simulink model "Automatic_Movement"  (R2015a)
settings: Solver=ode45  StartTime=0.0  StopTime=inf  FixedStep=0.05  RelTol=1e-3
values from neighbouring files (symbols this model uses):
  a_1 = 10.2    [Parameters.m]
  a_2 = 13.1    [Parameters.m]
  a_3 = 5.5    [Parameters.m]
  a_4 = 17    [Parameters.m]
  a_5 = 16.5    [Parameters.m]
  b_1 = 0.243    [Parameters.m]
  b_2 = 0.175    [Parameters.m]
  b_3 = 0.14    [Parameters.m]
  b_4 = 0.14    [Parameters.m]
  b_5 = 0.15    [Parameters.m]
  k1_1 = 2*alpha-a_1    (= 13.8)    [Parameters.m]
  k1_2 = 2*alpha-a_2    (= 10.9)    [Parameters.m]
  k1_3 = 2*alpha-a_3    (= 18.5)    [Parameters.m]
  k1_4 = 2*alpha-a_4    (= 7)    [Parameters.m]
  k1_5 = 2*alpha-a_5    (= 7.5)    [Parameters.m]
  k2_1 = alpha^2-b_1*k1_1    (= 140.6466)    [Parameters.m]
  k2_2 = alpha^2-b_2*k1_2    (= 142.0925)    [Parameters.m]
  k2_3 = alpha^2-b_3*k1_3    (= 141.41)    [Parameters.m]
  k2_4 = alpha^2-b_4*k1_4    (= 143.02)    [Parameters.m]
  k2_5 = alpha^2-b_5*k1_5    (= 142.875)    [Parameters.m]
  Ts = 0.06    [Parameters.m]
  Va = 24    [Parameters.m]
undefined symbols (not defined in the file or in its folder): DiscIntNeverNeededParam, gray, none, strel, videoinput
libraries: simulink x33, arduino_io_lib x28, visiontextngfix x6, visionanalysis x6, visionmorphops x4, visionstatistics x2, visionsinks x2, imaqlib x1
(part 1 of 2)
settings Model: CovMetricSettings=dwe  CovHtmlReporting=off  covSaveCumulativeToWorkspaceVar=off  CovSaveSingleToWorkspaceVar=off  CovExternalEMLEnable=on  ExtModeTrigDuration=10000  Creator=Antonio  LastModifiedBy=Antonio
settings SolverCC: PositivePriorityOrder=on
settings DataIOCC: LimitDataPoints=off  SaveFormat=Dataset
settings DebuggingCC: SFUnexpectedBacktrackingDiag=error  SFNoUnconditionalDefaultTransitionDiag=error
settings HardwareCC: ProdBitPerPointer=64  ProdLargestAtomicFloat=Float  ProdIntDivRoundTo=Zero  ProdEndianess=LittleEndian  ProdHWDeviceType=Specified
settings ModelReferenceCC: PropagateSignalLabelsOutOfModel=on
settings RTWCC: SystemTargetFile=quarc_win64.tlc  TemplateMakefile=quarc_default_tmf  Description=QUARC Win64 Target
settings STFCustomTargetCC: TargetLibSuffix=.lib  TargetPreCompLibLocation=C:\PROGRA~3\QUARC\lib\2017a\win64\release  TargetLangStandard=C99 (ISO)  GenerateSampleERTMain=off  ConcurrentExecutionCompliant=on  ERTCustomFileBanners=off  SupportNonInlinedSFcns=on  SupportVariableSizeSignals=off  MATLABClassNameForMDSCustomization=Simulink.SoftwareTarget.GRTCustomization  GRTInterface=on  SystemTargetFile=quarc_win64.tlc
settings GRTTargetCC: TargetPreCompLibLocation=C:\PROGRA~3\QUARC\lib\2017a\win64\release  TargetLangStandard=C99 (ISO)  ParMdlRefBuildCompliant=off  CompOptLevelCompliant=off  GeneratePreprocessorConditionals=Use local settings  CombineOutputUpdateFcns=off  MatFileLogging=off  CPPClassGenCompliant=off  GRTInterface=on  ExtMode=on  ExtModeMexFile=quarc_comm

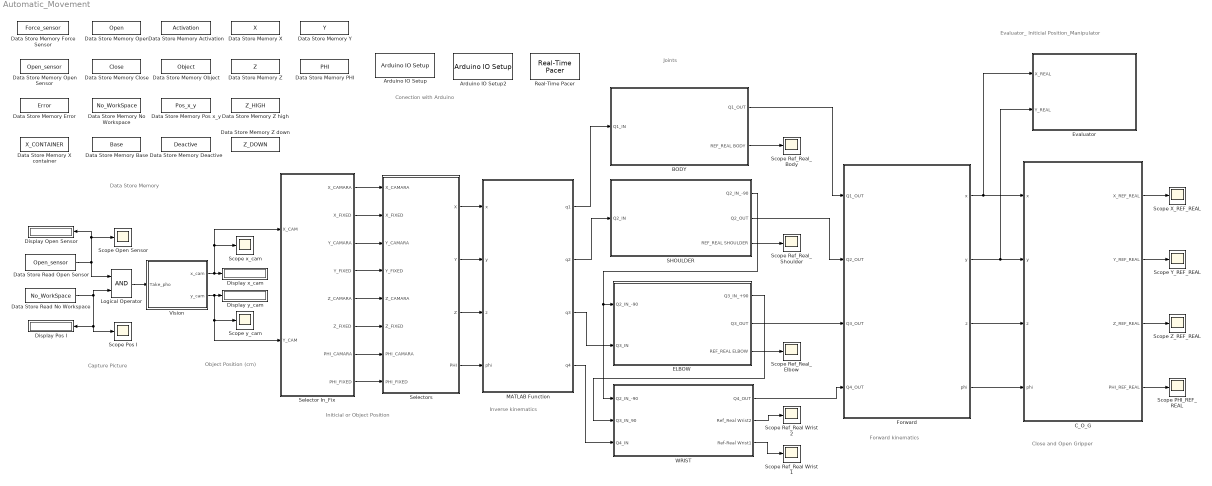
== system Automatic_Movement ==
  note: Close and Open Gripper
  note: Forward kinematics
  note: Joints
  note: Inverse kinematics
  note: Initicial or Object Position
  note: Evaluator_ Initicial Position_Manipulator
  note: Object Position
      | (cm)
  note: Capture Picture
  note: Data Store Memory
  note: Conection with Arduino
  Arduino IO Setup : arduino_io_lib/Arduino IO Setup  Priority=3  arduinoVar=Temporary arduino variable: Arduino1  workspaceVarName=a  comPort=COM3
  Arduino IO Setup2 : arduino_io_lib/Arduino IO Setup  Priority=3  arduinoVar=Temporary arduino variable: Arduino2  workspaceVarName=a  comPort=COM9
  BODY : Subsystem
  C_O_G : Subsystem
  Data Store Memory Base : DataStoreMemory  DataStoreName=Base  ReadBeforeWriteMsg=warning  WriteAfterWriteMsg=warning  WriteAfterReadMsg=warning  ShowAdditionalParam=off
  Data Store Memory Deactive : DataStoreMemory  DataStoreName=Deactive  ReadBeforeWriteMsg=warning  WriteAfterWriteMsg=warning  WriteAfterReadMsg=warning  ShowAdditionalParam=off
  Data Store Memory PHI : DataStoreMemory  DataStoreName=PHI  ReadBeforeWriteMsg=warning  WriteAfterWriteMsg=warning  WriteAfterReadMsg=warning  ShowAdditionalParam=off
  Data Store Memory Pos x_y : DataStoreMemory  DataStoreName=Pos_x_y  ReadBeforeWriteMsg=warning  WriteAfterWriteMsg=warning  WriteAfterReadMsg=warning  ShowAdditionalParam=off
  Data Store Memory Z : DataStoreMemory  DataStoreName=Z  ReadBeforeWriteMsg=warning  WriteAfterWriteMsg=warning  WriteAfterReadMsg=warning  ShowAdditionalParam=off
  Data Store Memory Z down : DataStoreMemory  DataStoreName=Z_DOWN  ReadBeforeWriteMsg=warning  WriteAfterWriteMsg=warning  WriteAfterReadMsg=warning  ShowAdditionalParam=off
  Data Store Memory Activation : DataStoreMemory  DataStoreName=Activation  ReadBeforeWriteMsg=warning  WriteAfterWriteMsg=warning  WriteAfterReadMsg=warning  ShowAdditionalParam=off
  "Data Store Memory Close " : DataStoreMemory  DataStoreName=Close  ReadBeforeWriteMsg=warning  WriteAfterWriteMsg=warning  WriteAfterReadMsg=warning  ShowAdditionalParam=off
  Data Store Memory Error : DataStoreMemory  DataStoreName=Error  ReadBeforeWriteMsg=warning  WriteAfterWriteMsg=warning  WriteAfterReadMsg=warning  ShowAdditionalParam=off
  Data Store Memory Force Sensor : DataStoreMemory  DataStoreName=Force_sensor  ReadBeforeWriteMsg=warning  WriteAfterWriteMsg=warning  WriteAfterReadMsg=warning  ShowAdditionalParam=off
  Data Store Memory No Workspace : DataStoreMemory  DataStoreName=No_WorkSpace  ReadBeforeWriteMsg=warning  WriteAfterWriteMsg=warning  WriteAfterReadMsg=warning  ShowAdditionalParam=off
  Data Store Memory Object : DataStoreMemory  DataStoreName=Object  ReadBeforeWriteMsg=warning  WriteAfterWriteMsg=warning  WriteAfterReadMsg=warning  ShowAdditionalParam=off
  Data Store Memory Open : DataStoreMemory  DataStoreName=Open  ReadBeforeWriteMsg=warning  WriteAfterWriteMsg=warning  WriteAfterReadMsg=warning  ShowAdditionalParam=off
  Data Store Memory Open Sensor : DataStoreMemory  DataStoreName=Open_sensor  ReadBeforeWriteMsg=warning  WriteAfterWriteMsg=warning  WriteAfterReadMsg=warning  ShowAdditionalParam=off
  Data Store Memory X : DataStoreMemory  DataStoreName=X  ReadBeforeWriteMsg=warning  WriteAfterWriteMsg=warning  WriteAfterReadMsg=warning  ShowAdditionalParam=off
  Data Store Memory X container : DataStoreMemory  DataStoreName=X_CONTAINER  ReadBeforeWriteMsg=warning  WriteAfterWriteMsg=warning  WriteAfterReadMsg=warning  ShowAdditionalParam=off
  Data Store Memory Y : DataStoreMemory  DataStoreName=Y  ReadBeforeWriteMsg=warning  WriteAfterWriteMsg=warning  WriteAfterReadMsg=warning  ShowAdditionalParam=off
  Data Store Memory Z high : DataStoreMemory  DataStoreName=Z_HIGH  ReadBeforeWriteMsg=warning  WriteAfterWriteMsg=warning  WriteAfterReadMsg=warning  ShowAdditionalParam=off
  Data Store Read No Workspace : DataStoreRead  DataStoreName=No_WorkSpace  SampleTime=Ts
  Data Store Read Open Sensor : DataStoreRead  DataStoreName=Open_sensor  SampleTime=Ts
  Display Open Sensor : Display
  Display Pos I : Display
  Display x_cam : Display
  Display y_cam : Display
  ELBOW : Subsystem
  Evaluator : Subsystem
  Forward : Subsystem
  Logical Operator : Logic  AllPortsSameDT=off  OutDataTypeStr=boolean
  "MATLAB Function " : MATLAB Function  TreatAsAtomicUnit=on
      settings: PermitHierarchicalResolution=ParametersOnly
  Real-Time Pacer : arduino_io_lib/Real-Time Pacer  simTimePerRealTime=1
  "SHOULDER " : Subsystem
  Scope PHI_REF_REAL : Scope
      settings: TimeRange=auto  MaxDataPoints=5000  SaveToWorkspace=off  SaveName=ScopeData4  YMin=-10  YMax=10  SampleTime=-1
  Scope Ref_Real Wrist 1 : Scope
      settings: TimeRange=auto  MaxDataPoints=5000  SaveName=c  YMin=-0.01172  YMax=0.0013  SampleTime=-1
  Scope Ref_Real Wrist 2 : Scope
      settings: TimeRange=auto  MaxDataPoints=5000  SaveName=b  YMin=-0.00213  YMax=0.00024  SampleTime=-1
  Scope Ref_Real_Body : Scope
      settings: TimeRange=auto  MaxDataPoints=5000  SaveName=base  YMin=-0.17745  YMax=1.59701  SampleTime=-1
  Scope Ref_Real_Elbow : Scope
      settings: TimeRange=auto  MaxDataPoints=5000  SaveName=codo  YMin=-0.0889  YMax=0.80013  SampleTime=-1
  Scope Ref_Real_Shoulder : Scope
      settings: TimeRange=auto  MaxDataPoints=5000  SaveName=hombro  YMin=-0.7513  YMax=0.08348  SampleTime=-1
  Scope X_REF_REAL : Scope
      settings: TimeRange=auto  MaxDataPoints=5000  SaveToWorkspace=off  YMin=-10  YMax=10  SampleTime=-1
  Scope Y_REF_REAL : Scope
      settings: TimeRange=auto  MaxDataPoints=5000  SaveToWorkspace=off  SaveName=ScopeData2  YMin=-10  YMax=10  SampleTime=-1
  Scope Z_REF_REAL : Scope
      settings: TimeRange=auto  MaxDataPoints=5000  SaveToWorkspace=off  SaveName=ScopeData3  YMin=-10  YMax=10  SampleTime=-1
  Scope Open Sensor : Scope
      settings: TimeRange=100  MaxDataPoints=5000  SaveToWorkspace=off  SaveName=ScopeData2  YMin=-0.125  YMax=1.125  SampleTime=-1
  Scope Pos I : Scope
      settings: TimeRange=100  MaxDataPoints=5000  SaveToWorkspace=off  YMin=-0.125  YMax=1.125  SampleTime=-1
  Scope x_cam : Scope
      settings: TimeRange=100  MaxDataPoints=5000  SaveToWorkspace=off  SaveName=ScopeData4  YMin=3.92736  YMax=4.48639  SampleTime=-1
  Scope y_cam : Scope
      settings: TimeRange=100  MaxDataPoints=5000  SaveToWorkspace=off  SaveName=ScopeData5  YMin=-1.15286  YMax=10.37571  SampleTime=-1
  Selector In_Fix : Subsystem
  Selectors : Subsystem
  Vision : Subsystem
  WRIST : Subsystem
  wires:
  "MATLAB Function "/2(q2) -> "SHOULDER "/1(Q2_IN)
  "SHOULDER "/1("Q2_IN_-90 ") -> WRIST/1(Q2_IN_-90), ELBOW/1(Q2_IN_-90)
  "MATLAB Function "/3(q3) -> ELBOW/2(Q3_IN)
  "MATLAB Function "/4(q4) -> WRIST/3(Q4_IN)
  "MATLAB Function "/1(q1) -> BODY/1(Q1_IN)
  ELBOW/1(Q3_IN_+90) -> WRIST/2("Q3_IN_90 ")
  "SHOULDER "/3(REF_REAL SHOULDER) -> Scope Ref_Real_Shoulder/1
  BODY/2(REF_REAL BODY) -> Scope Ref_Real_Body/1
  ELBOW/3(REF_REAL ELBOW) -> Scope Ref_Real_Elbow/1
  WRIST/3(Ref-Real Wrist1) -> Scope Ref_Real Wrist 1/1
  WRIST/2(Ref_Real Wrist2) -> Scope Ref_Real Wrist 2/1
  BODY/1(Q1_OUT) -> Forward/1(Q1_OUT)
  "SHOULDER "/2(Q2_OUT) -> Forward/2(Q2_OUT)
  WRIST/1(Q4_OUT) -> Forward/4(Q4_OUT)
  Forward/3(z) -> C_O_G/3(z)
  Forward/4(phi) -> C_O_G/4(phi)
  Selector In_Fix/8(PHI_FIXED) -> Selectors/8(PHI_FIXED)
  Selector In_Fix/7(PHI_CAMARA) -> Selectors/7(PHI_CAMARA)
  Selector In_Fix/2(X_FIXED) -> Selectors/2(X_FIXED)
  Selector In_Fix/5(Z_CAMARA) -> Selectors/5(Z_CAMARA)
  Selector In_Fix/3(Y_CAMARA) -> Selectors/3(Y_CAMARA)
  Selector In_Fix/4(Y_FIXED) -> Selectors/4(Y_FIXED)
  Selector In_Fix/1(X_CAMARA) -> Selectors/1(X_CAMARA)
  Selector In_Fix/6(Z_FIXED) -> Selectors/6(Z_FIXED)
  Forward/1(x) -> C_O_G/1(x), Evaluator/1(X_REAL)
  Forward/2(y) -> C_O_G/2(y), Evaluator/2(Y_REAL)
  Logical Operator/1 -> Vision/1(Take_pho)
  Data Store Read Open Sensor/1 -> Display Open Sensor/1, Scope Open Sensor/1, Logical Operator/1
  Vision/2(y_cam) -> Display y_cam/1, Selector In_Fix/2(Y_CAM), Scope y_cam/1
  Data Store Read No Workspace/1 -> Logical Operator/2, Display Pos I/1, Scope Pos I/1
  Vision/1(x_cam) -> Selector In_Fix/1(X_CAM), Scope x_cam/1, Display x_cam/1
  Selectors/1("X ") -> "MATLAB Function "/1(x)
  Selectors/4(PHI) -> "MATLAB Function "/4(phi)
  Selectors/3(Z) -> "MATLAB Function "/3(z)
  Selectors/2(Y) -> "MATLAB Function "/2(y)
  ELBOW/2(Q3_OUT) -> Forward/3(Q3_OUT)
  C_O_G/1(X_REF_REAL) -> Scope X_REF_REAL/1
  C_O_G/3(Z_REF_REAL) -> Scope Z_REF_REAL/1
  C_O_G/2(Y_REF_REAL) -> Scope Y_REF_REAL/1
  C_O_G/4(PHI_REF_REAL) -> Scope PHI_REF_REAL/1

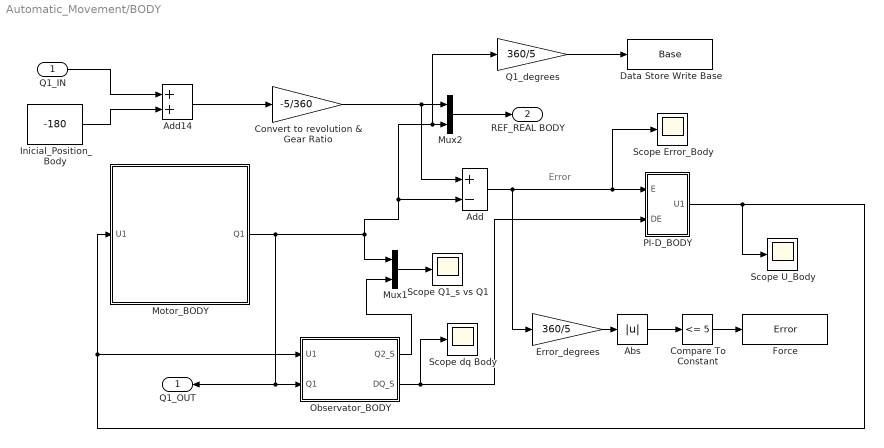
== system Automatic_Movement/BODY ==
  note: Error
  Q1_IN : Inport
  " Scope dq Body" : Scope
      settings: TimeRange=auto  MaxDataPoints=5000  SaveName=dq_cintura  YMin=-0.73219  YMax=0.72449  SampleTime=-1
  Abs : Abs
  Add : Sum  Inputs=+-
  Add14 : Sum
  Compare To Constant : simulink/Logic and Bit Operations/Compare To Constant  relop=<=  const=5  OutDataTypeStr=boolean
  "Convert to revolution & Gear Ratio " : Gain  Gain=-5/360
  Data Store Write Base : DataStoreWrite  DataStoreName=Base  SampleTime=Ts
  Error_degrees : Gain  Gain=360/5
  Force : DataStoreWrite  DataStoreName=Error  SampleTime=Ts
  Inicial_Position_Body : Constant  Value=-180  SampleTime=Ts
  Motor_BODY : Subsystem
  Mux1 : Mux  Inputs=2
  Mux2 : Mux  Inputs=2
  Observator_BODY : Subsystem
  PI-D_BODY : Subsystem
  Q1_degrees : Gain  Gain=360/5
  "Scope Error_Body " : Scope
      settings: TimeRange=auto  MaxDataPoints=5000  SaveName=e_cintura  YMin=-0.06288  YMax=0.53501  SampleTime=-1
  Scope Q1_s vs Q1 : Scope
      settings: TimeRange=100  MaxDataPoints=5000  SaveToWorkspace=off  YMin=-0.02657  YMax=0.23915  SampleTime=-1  DataFormat=Array
  "Scope U_Body " : Scope
      settings: TimeRange=auto  MaxDataPoints=5000  SaveName=u_cintura  YMin=-18.237  YMax=28.693  SampleTime=-1
  Q1_OUT : Outport
  REF_REAL BODY : Outport  Port=2
  wires:
  PI-D_BODY/1(U1) -> "Scope U_Body "/1, Motor_BODY/1(U1), Observator_BODY/1(U1)
  Observator_BODY/2(DQ_S) -> PI-D_BODY/2(DE), " Scope dq Body"/1
  Mux2/1 -> REF_REAL BODY/1
  "Convert to revolution & Gear Ratio "/1 -> Mux2/1, Add/1
  Error_degrees/1 -> Abs/1
  Motor_BODY/1(Q1) -> Add/2, Q1_degrees/1, Mux2/2, Mux1/1, Q1_OUT/1, Observator_BODY/2(Q1)
  Add/1 -> "Scope Error_Body "/1, PI-D_BODY/1(E), Error_degrees/1
  Mux1/1 -> Scope Q1_s vs Q1/1
  Observator_BODY/1(Q2_S) -> Mux1/2
  Add14/1 -> "Convert to revolution & Gear Ratio "/1
  Q1_IN/1 -> Add14/1
  Inicial_Position_Body/1 -> Add14/2
  Abs/1 -> Compare To Constant/1
  Compare To Constant/1 -> Force/1
  Q1_degrees/1 -> Data Store Write Base/1

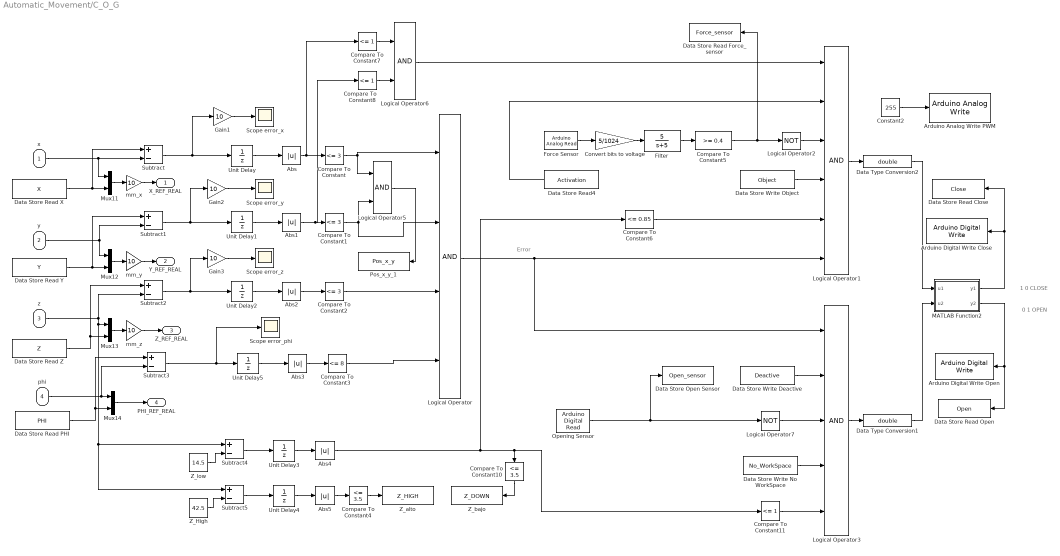
== system Automatic_Movement/C_O_G ==
  note: Error
  note: 0 1 OPEN
  note: 1 0 CLOSE
  x : Inport
  y : Inport  Port=2
  z : Inport  Port=3
  phi : Inport  Port=4
  Abs{,1..5} (6 alike) : Abs  ZeroCross=off
  Arduino Analog Write PWM : arduino_io_lib/Arduino Analog Write  arduinoVar=Temporary arduino variable: Arduino1  arduinoPin=9  T=Ts
  Arduino Digital Write Open : arduino_io_lib/Arduino Digital Write  arduinoVar=Temporary arduino variable: Arduino1  arduinoPin=7  T=Ts
  Arduino Digital Write Close : arduino_io_lib/Arduino Digital Write  arduinoVar=Temporary arduino variable: Arduino1  arduinoPin=6  T=Ts
  Compare To Constant : simulink/Logic and Bit Operations/Compare To Constant  relop=<=  const=3  OutDataTypeStr=boolean  ZeroCross=off
  Compare To Constant1 : simulink/Logic and Bit Operations/Compare To Constant  relop=<=  const=3  OutDataTypeStr=boolean  ZeroCross=off
  Compare To Constant10 : simulink/Logic and Bit Operations/Compare To Constant  relop=<=  const=3.5  OutDataTypeStr=boolean  ZeroCross=off
  Compare To Constant11 : simulink/Logic and Bit Operations/Compare To Constant  relop=<=  const=1  OutDataTypeStr=boolean  ZeroCross=off
  Compare To Constant2 : simulink/Logic and Bit Operations/Compare To Constant  relop=<=  const=3  OutDataTypeStr=boolean
  Compare To Constant3 : simulink/Logic and Bit Operations/Compare To Constant  relop=<=  const=8  OutDataTypeStr=boolean  ZeroCross=off
  Compare To Constant4 : simulink/Logic and Bit Operations/Compare To Constant  relop=<=  const=3.5  OutDataTypeStr=boolean  ZeroCross=off
  Compare To Constant5 : simulink/Logic and Bit Operations/Compare To Constant  relop=>=  const=0.4  OutDataTypeStr=boolean  ZeroCross=off
  Compare To Constant6 : simulink/Logic and Bit Operations/Compare To Constant  relop=<=  const=0.85  OutDataTypeStr=boolean  ZeroCross=off
  Compare To Constant7 : simulink/Logic and Bit Operations/Compare To Constant  relop=<=  const=1  OutDataTypeStr=boolean  ZeroCross=off
  Compare To Constant8 : simulink/Logic and Bit Operations/Compare To Constant  relop=<=  const=1  OutDataTypeStr=boolean  ZeroCross=off
  Constant2 : Constant  Value=255
  Convert bits to voltage : Gain  Gain=5/1024
  Data Store Open Sensor : DataStoreWrite  DataStoreName=Open_sensor  SampleTime=Ts
  Data Store Read PHI : DataStoreRead  DataStoreName=PHI  SampleTime=Ts
  Data Store Read X : DataStoreRead  DataStoreName=X  SampleTime=Ts
  Data Store Read Y : DataStoreRead  DataStoreName=Y  SampleTime=Ts
  Data Store Read Z : DataStoreRead  DataStoreName=Z  SampleTime=Ts
  Data Store Read4 : DataStoreRead  DataStoreName=Activation  SampleTime=Ts
  Data Store Write Deactive : DataStoreRead  DataStoreName=Deactive  SampleTime=Ts
  Data Store Write No WorkSpace : DataStoreRead  DataStoreName=No_WorkSpace
  Data Store Write Object : DataStoreRead  DataStoreName=Object  SampleTime=Ts
  Data Store Read Close : DataStoreWrite  DataStoreName=Close  SampleTime=Ts
  Data Store Read Force_sensor : DataStoreWrite  DataStoreName=Force_sensor  SampleTime=Ts
  Data Store Read Open : DataStoreWrite  DataStoreName=Open  SampleTime=Ts
  Data Type Conversion1 : DataTypeConversion  OutDataTypeStr=double
  Data Type Conversion2 : DataTypeConversion  OutDataTypeStr=double
  Filter : TransferFcn  Numerator=[5]  Denominator=[1 5]
  Force Sensor : arduino_io_lib/Arduino Analog Read  arduinoVar=Temporary arduino variable: Arduino1  arduinoPin=0  T=Ts
  Gain1 : Gain  Gain=10
  Gain2 : Gain  Gain=10
  Gain3 : Gain  Gain=10
  Logical Operator : Logic  Inputs=4  AllPortsSameDT=off  OutDataTypeStr=boolean
  Logical Operator1 : Logic  Inputs=6  AllPortsSameDT=off  OutDataTypeStr=boolean
  Logical Operator2 : Logic  Operator=NOT  AllPortsSameDT=off  OutDataTypeStr=boolean
  Logical Operator3 : Logic  Inputs=5  AllPortsSameDT=off  OutDataTypeStr=boolean
  Logical Operator5 : Logic  AllPortsSameDT=off  OutDataTypeStr=boolean
  Logical Operator6 : Logic  AllPortsSameDT=off  OutDataTypeStr=boolean
  Logical Operator7 : Logic  Operator=NOT  AllPortsSameDT=off  OutDataTypeStr=boolean
  MATLAB Function2 : MATLAB Function  TreatAsAtomicUnit=on
      settings: PermitHierarchicalResolution=ParametersOnly
  Mux{11..14} (4 alike) : Mux  Inputs=2
  Opening Sensor : arduino_io_lib/Arduino Digital Read  arduinoVar=Temporary arduino variable: Arduino1  arduinoPin=34  T=Ts
  "Pos_x_y_1 " : DataStoreWrite  DataStoreName=Pos_x_y  SampleTime=Ts
  "Scope error_phi " : Scope
      settings: TimeRange=auto  MaxDataPoints=5000  SaveName=e_phi  YMin=89.82624  YMax=91.56383  SampleTime=-1
  "Scope error_x " : Scope
      settings: TimeRange=auto  MaxDataPoints=5000  SaveName=e_x  YMin=-74.61173  YMax=252.73464  SampleTime=-1
  "Scope error_y " : Scope
      settings: TimeRange=auto  MaxDataPoints=5000  SaveName=e_y  YMin=-68.99271  YMax=196.55475  SampleTime=-1
  Scope error_z : Scope
      settings: TimeRange=auto  MaxDataPoints=5000  SaveName=e_z  YMin=-538.89547  YMax=350.0592  SampleTime=-1
  Subtract{,1..5} (6 alike) : Sum  Inputs=+-
  Unit Delay{,1..5} (6 alike) : UnitDelay  SampleTime=Ts
  Z_High : Constant  Value=42.5
  "Z_alto " : DataStoreWrite  DataStoreName=Z_HIGH  SampleTime=Ts
  Z_bajo : DataStoreWrite  DataStoreName=Z_DOWN  SampleTime=Ts
  Z_low : Constant  Value=14.5
  mm_x : Gain  Gain=10
  mm_y : Gain  Gain=10
  mm_z : Gain  Gain=10
  X_REF_REAL : Outport
  Y_REF_REAL : Outport  Port=2
  Z_REF_REAL : Outport  Port=3
  PHI_REF_REAL : Outport  Port=4
  wires:
  Data Store Read4/1 -> Logical Operator1/2
  Data Store Read X/1 -> Mux11/2, Subtract/1
  x/1 -> Mux11/1, Subtract/2
  y/1 -> Mux12/1, Subtract1/2
  phi/1 -> Subtract3/2, Mux14/1
  Abs/1 -> Compare To Constant/1, Compare To Constant7/1
  Compare To Constant1/1 -> Logical Operator/2, Logical Operator5/2
  Abs2/1 -> Compare To Constant2/1
  Compare To Constant3/1 -> Logical Operator/4
  Compare To Constant/1 -> Logical Operator/1, Logical Operator5/1
  Mux13/1 -> mm_z/1
  Compare To Constant2/1 -> Logical Operator/3
  Mux11/1 -> mm_x/1
  Mux12/1 -> mm_y/1
  Abs3/1 -> Compare To Constant3/1
  Opening Sensor/1 -> Logical Operator7/1, Data Store Open Sensor/1
  Logical Operator3/1 -> Data Type Conversion1/1
  Force Sensor/1 -> Convert bits to voltage/1
  Compare To Constant5/1 -> Logical Operator2/1, Data Store Read Force_sensor/1
  Logical Operator1/1 -> Data Type Conversion2/1
  Subtract1/1 -> Unit Delay1/1, Gain2/1
  Subtract/1 -> Unit Delay/1, Gain1/1
  Subtract2/1 -> Unit Delay2/1, Gain3/1
  Logical Operator2/1 -> Logical Operator1/3
  Data Type Conversion2/1 -> MATLAB Function2/1(u1)
  Data Store Write Deactive/1 -> Logical Operator3/2
  Logical Operator7/1 -> Logical Operator3/3
  Data Type Conversion1/1 -> MATLAB Function2/2(u2)
  Data Store Read PHI/1 -> Mux14/2, Subtract3/1
  Data Store Read Z/1 -> Mux13/2, Subtract2/1
  Data Store Read Y/1 -> Mux12/2, Subtract1/1
  Data Store Write Object/1 -> Logical Operator1/4
  Subtract4/1 -> Unit Delay3/1
  Z_low/1 -> Subtract4/2
  Logical Operator5/1 -> "Pos_x_y_1 "/1
  Z_High/1 -> Subtract5/2
  Compare To Constant4/1 -> "Z_alto "/1
  Subtract5/1 -> Unit Delay4/1
  Abs5/1 -> Compare To Constant4/1
  z/1 -> Subtract5/1, Subtract4/1, Mux13/1, Subtract2/2
  Data Store Write No WorkSpace/1 -> Logical Operator3/4
  Constant2/1 -> Arduino Analog Write PWM/1
  Convert bits to voltage/1 -> Filter/1
  Logical Operator/1 -> Logical Operator3/1, Logical Operator1/6
  MATLAB Function2/1(y1) -> Arduino Digital Write Close/1, Data Store Read Close/1
  MATLAB Function2/2(y2) -> Arduino Digital Write Open/1, Data Store Read Open/1
  Abs1/1 -> Compare To Constant1/1, Compare To Constant8/1
  Compare To Constant7/1 -> Logical Operator6/1
  Compare To Constant8/1 -> Logical Operator6/2
  Unit Delay/1 -> Abs/1
  Unit Delay1/1 -> Abs1/1
  Unit Delay2/1 -> Abs2/1
  Unit Delay3/1 -> Abs4/1
  Unit Delay4/1 -> Abs5/1
  Unit Delay5/1 -> Abs3/1
  Filter/1 -> Compare To Constant5/1
  Abs4/1 -> Compare To Constant6/1, Compare To Constant10/1, Compare To Constant11/1
  Compare To Constant10/1 -> Z_bajo/1
  Compare To Constant6/1 -> Logical Operator1/5
  Compare To Constant11/1 -> Logical Operator3/5
  Gain1/1 -> "Scope error_x "/1
  Gain2/1 -> "Scope error_y "/1
  Gain3/1 -> Scope error_z/1
  Subtract3/1 -> "Scope error_phi "/1, Unit Delay5/1
  mm_y/1 -> Y_REF_REAL/1
  mm_x/1 -> X_REF_REAL/1
  mm_z/1 -> Z_REF_REAL/1
  Mux14/1 -> PHI_REF_REAL/1
  Logical Operator6/1 -> Logical Operator1/1

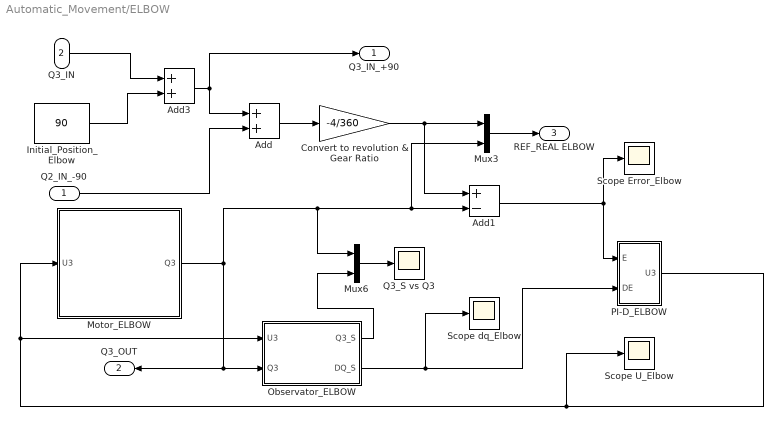
== system Automatic_Movement/ELBOW ==
  Q2_IN_-90 : Inport
  Q3_IN : Inport  Port=2
  Add : Sum
  Add1 : Sum  Inputs=+-
  Add3 : Sum
  Convert to revolution & Gear Ratio : Gain  Gain=-4/360
  Initial_Position_Elbow : Constant  Value=90  SampleTime=Ts
  Motor_ELBOW : Subsystem
  Mux3 : Mux  Inputs=2
  Mux6 : Mux  Inputs=2
  Observator_ELBOW : Subsystem
  PI-D_ELBOW : Subsystem
  Q3_S vs Q3 : Scope
      settings: TimeRange=100  MaxDataPoints=5000  SaveToWorkspace=off  SaveName=ScopeData4  YMin=-0.09176  YMax=0.82585  SampleTime=-1  DataFormat=Array
  Scope Error_Elbow : Scope
      settings: TimeRange=auto  MaxDataPoints=5000  SaveName=e_codo  YMin=-0.09784  YMax=0.79717  SampleTime=-1
  Scope U_Elbow : Scope
      settings: TimeRange=auto  MaxDataPoints=5000  SaveName=u_codo  YMin=-30.00000  YMax=30.00000  SampleTime=-1
  Scope dq_Elbow : Scope
      settings: TimeRange=auto  MaxDataPoints=5000  SaveName=dq_codo  YMin=-0.07154  YMax=0.22276  SampleTime=-1
  Q3_IN_+90 : Outport
  Q3_OUT : Outport  Port=2
  REF_REAL ELBOW : Outport  Port=3
  wires:
  Q2_IN_-90/1 -> Add/2
  PI-D_ELBOW/1(U3) -> Motor_ELBOW/1(U3), Observator_ELBOW/1(U3), Scope U_Elbow/1
  Observator_ELBOW/2(DQ_S) -> Scope dq_Elbow/1, PI-D_ELBOW/2(DE)
  Convert to revolution & Gear Ratio/1 -> Mux3/1, Add1/1
  Mux3/1 -> REF_REAL ELBOW/1
  Motor_ELBOW/1(Q3) -> Mux3/2, Add1/2, Mux6/1, Observator_ELBOW/2(Q3), Q3_OUT/1
  Add/1 -> Convert to revolution & Gear Ratio/1
  Add1/1 -> Scope Error_Elbow/1, PI-D_ELBOW/1(E)
  Add3/1 -> Q3_IN_+90/1, Add/1
  Mux6/1 -> Q3_S vs Q3/1
  Observator_ELBOW/1(Q3_S) -> Mux6/2
  Q3_IN/1 -> Add3/1
  Initial_Position_Elbow/1 -> Add3/2

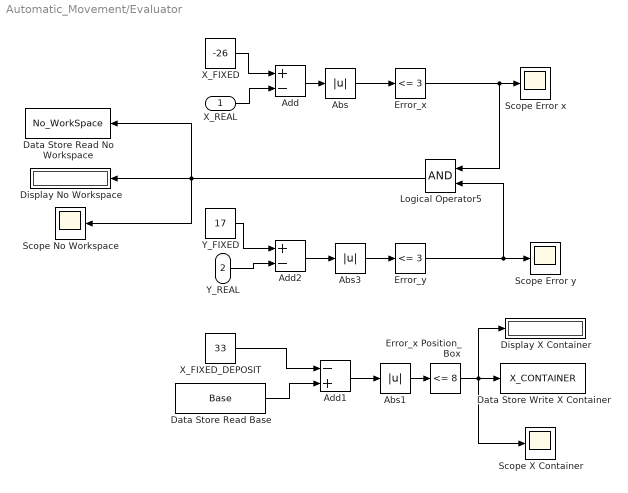
== system Automatic_Movement/Evaluator ==
  X_REAL : Inport
  Y_REAL : Inport  Port=2
  Abs : Abs  ZeroCross=off
  Abs1 : Abs  ZeroCross=off
  Abs3 : Abs  ZeroCross=off
  Add : Sum  Inputs=+-
  Add1 : Sum  Inputs=-+
  Add2 : Sum  Inputs=+-
  Data Store Read Base : DataStoreRead  DataStoreName=Base  SampleTime=Ts
  Data Store Read No Workspace : DataStoreWrite  DataStoreName=No_WorkSpace  SampleTime=Ts
  Data Store Write X Container : DataStoreWrite  DataStoreName=X_CONTAINER  SampleTime=Ts
  Display No Workspace : Display
  Display X Container : Display
  Error_x : simulink/Logic and Bit Operations/Compare To Constant  relop=<=  const=3  OutDataTypeStr=boolean  ZeroCross=off
  Error_x Position_Box : simulink/Logic and Bit Operations/Compare To Constant  relop=<=  const=8  OutDataTypeStr=boolean  ZeroCross=off
  Error_y : simulink/Logic and Bit Operations/Compare To Constant  relop=<=  const=3  OutDataTypeStr=boolean  ZeroCross=off
  Logical Operator5 : Logic  AllPortsSameDT=off  OutDataTypeStr=boolean
  Scope Error x : Scope
      settings: TimeRange=100  MaxDataPoints=5000  SaveToWorkspace=off  YMin=-0.125  YMax=1.125  SampleTime=-1
  Scope Error y : Scope
      settings: TimeRange=100  MaxDataPoints=5000  SaveToWorkspace=off  SaveName=ScopeData2  YMin=-0.125  YMax=1.125  SampleTime=-1
  Scope No Workspace : Scope
      settings: TimeRange=100  MaxDataPoints=5000  SaveToWorkspace=off  SaveName=ScopeData5  YMin=-0.125  YMax=1.125  SampleTime=-1
  Scope X Container : Scope
      settings: TimeRange=100  MaxDataPoints=5000  SaveToWorkspace=off  YMin=-0.125  YMax=1.125  SampleTime=-1
  X_FIXED : Constant  Value=-26
  X_FIXED_DEPOSIT : Constant  Value=33
  Y_FIXED : Constant  Value=17
  wires:
  Abs/1 -> Error_x/1
  Abs3/1 -> Error_y/1
  X_FIXED/1 -> Add/1
  Error_x/1 -> Scope Error x/1, Logical Operator5/1
  Add/1 -> Abs/1
  Error_y/1 -> Scope Error y/1, Logical Operator5/2
  Add2/1 -> Abs3/1
  X_REAL/1 -> Add/2
  Y_REAL/1 -> Add2/2
  Y_FIXED/1 -> Add2/1
  Logical Operator5/1 -> Data Store Read No Workspace/1, Scope No Workspace/1, Display No Workspace/1
  X_FIXED_DEPOSIT/1 -> Add1/1
  Data Store Read Base/1 -> Add1/2
  Abs1/1 -> Error_x Position_Box/1
  Add1/1 -> Abs1/1
  Error_x Position_Box/1 -> Display X Container/1, Scope X Container/1, Data Store Write X Container/1

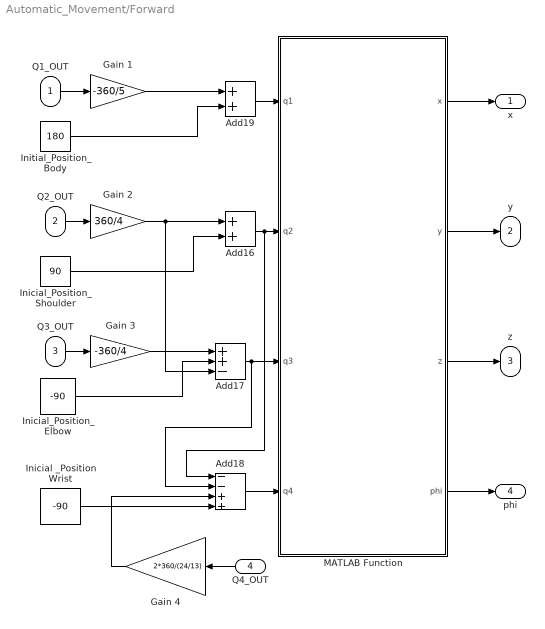
== system Automatic_Movement/Forward ==
  Q1_OUT : Inport
  Q2_OUT : Inport  Port=2
  Q3_OUT : Inport  Port=3
  Q4_OUT : Inport  Port=4
  Add16 : Sum
  Add17 : Sum  Inputs=++-
  Add18 : Sum  Inputs=--++
  Add19 : Sum
  "Gain 1 " : Gain  Gain=-360/5
  Gain 2 : Gain  Gain=360/4
  Gain 3 : Gain  Gain=-360/4
  Gain 4 : Gain  Gain=2*360/(24/13)
  Inicial _Position Wrist : Constant  Value=-90
  Inicial_Position_Elbow : Constant  Value=-90
  Inicial_Position_Shoulder : Constant  Value=90
  Initial_Position_Body : Constant  Value=180
  MATLAB Function : MATLAB Function  TreatAsAtomicUnit=on
      settings: PermitHierarchicalResolution=ParametersOnly
  x : Outport
  y : Outport  Port=2
  z : Outport  Port=3
  phi : Outport  Port=4
  wires:
  Add19/1 -> MATLAB Function/1(q1)
  Inicial _Position Wrist/1 -> Add18/4
  Add16/1 -> Add18/1, MATLAB Function/2(q2)
  Initial_Position_Body/1 -> Add19/2
  Gain 3/1 -> Add17/1
  "Gain 1 "/1 -> Add19/1
  Gain 2/1 -> Add17/3, Add16/1
  Add17/1 -> Add18/2, MATLAB Function/3(q3)
  Q4_OUT/1 -> Gain 4/1
  MATLAB Function/4(phi) -> phi/1
  MATLAB Function/2(y) -> y/1
  Inicial_Position_Elbow/1 -> Add17/2
  MATLAB Function/1(x) -> x/1
  MATLAB Function/3(z) -> z/1
  Add18/1 -> MATLAB Function/4(q4)
  Gain 4/1 -> Add18/3
  Inicial_Position_Shoulder/1 -> Add16/2
  Q1_OUT/1 -> "Gain 1 "/1
  Q3_OUT/1 -> Gain 3/1
  Q2_OUT/1 -> Gain 2/1

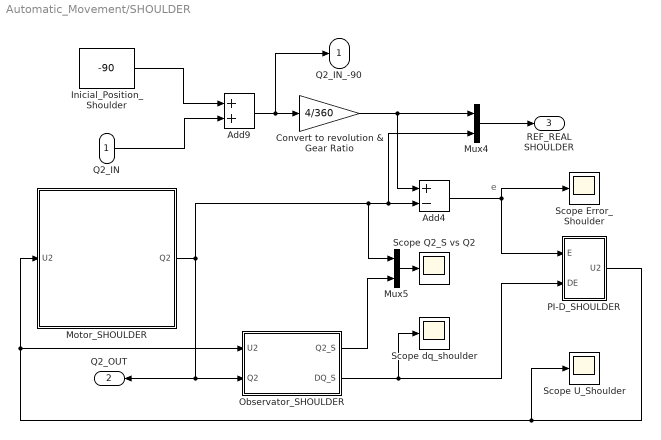
== system Automatic_Movement/SHOULDER  ==
  note: e
  Q2_IN : Inport
  Add4 : Sum  Inputs=+-
  Add9 : Sum
  Convert to revolution & Gear Ratio : Gain  Gain=4/360
  Inicial_Position_Shoulder : Constant  Value=-90  SampleTime=Ts
  "Motor_SHOULDER " : Subsystem
  Mux4 : Mux  Inputs=2
  Mux5 : Mux  Inputs=2
  Observator_SHOULDER : Subsystem
  PI-D_SHOULDER : Subsystem
  Scope Error_Shoulder : Scope
      settings: TimeRange=auto  MaxDataPoints=5000  SaveName=e_hombro  YMin=-0.51149  YMax=0.18642  SampleTime=-1
  Scope Q2_S vs Q2 : Scope
      settings: TimeRange=100  MaxDataPoints=5000  SaveToWorkspace=off  SaveName=ScopeData3  YMin=-0.80566  YMax=0.08952  SampleTime=-1  DataFormat=Array
  "Scope U_Shoulder " : Scope
      settings: TimeRange=auto  MaxDataPoints=5000  SaveName=u_hombro  YMin=-30.00000  YMax=30.00000  SampleTime=-1
  Scope dq_shoulder : Scope
      settings: TimeRange=auto  MaxDataPoints=5000  SaveName=dq_hombro  YMin=-0.19759  YMax=0.09122  SampleTime=-1
  "Q2_IN_-90 " : Outport
  Q2_OUT : Outport  Port=2
  REF_REAL SHOULDER : Outport  Port=3
  wires:
  Add4/1 -> Scope Error_Shoulder/1, PI-D_SHOULDER/1(E)
  PI-D_SHOULDER/1(U2) -> Observator_SHOULDER/1(U2), "Motor_SHOULDER "/1(U2), "Scope U_Shoulder "/1
  Observator_SHOULDER/2(DQ_S) -> Scope dq_shoulder/1, PI-D_SHOULDER/2(DE)
  Convert to revolution & Gear Ratio/1 -> Add4/1, Mux4/1
  Mux4/1 -> REF_REAL SHOULDER/1
  Observator_SHOULDER/1(Q2_S) -> Mux5/2
  Mux5/1 -> Scope Q2_S vs Q2/1
  "Motor_SHOULDER "/1(Q2) -> Observator_SHOULDER/2(Q2), Q2_OUT/1, Mux5/1, Add4/2, Mux4/2
  Add9/1 -> "Q2_IN_-90 "/1, Convert to revolution & Gear Ratio/1
  Q2_IN/1 -> Add9/2
  Inicial_Position_Shoulder/1 -> Add9/1

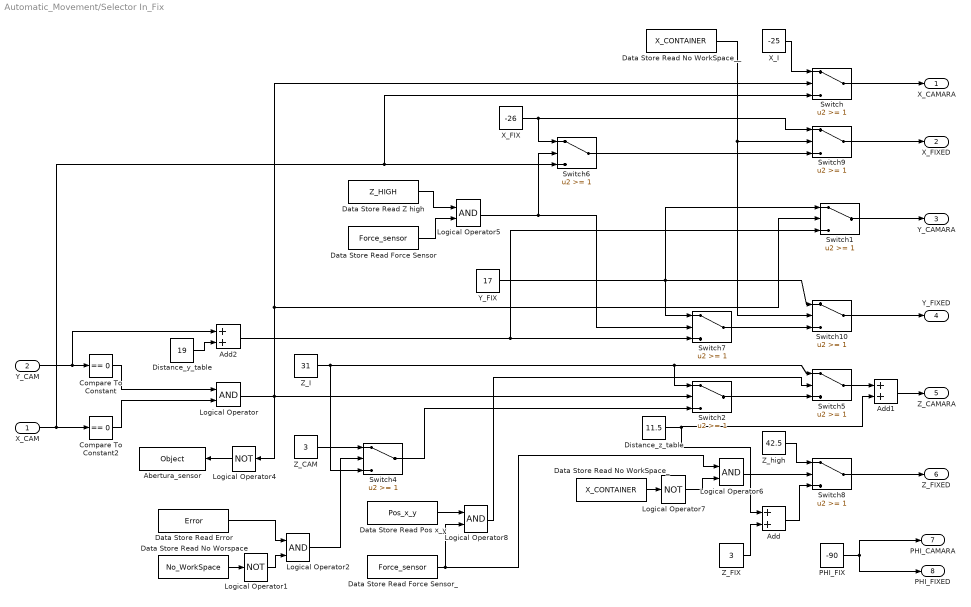
== system Automatic_Movement/Selector In_Fix ==
  X_CAM : Inport
  Y_CAM : Inport  Port=2
  Abertura_sensor : DataStoreWrite  DataStoreName=Object  SampleTime=Ts
  Add : Sum
  Add1 : Sum
  Add2 : Sum
  Compare To Constant : simulink/Logic and Bit Operations/Compare To Constant  relop===  const=0  OutDataTypeStr=boolean  ZeroCross=off
  Compare To Constant2 : simulink/Logic and Bit Operations/Compare To Constant  relop===  const=0  OutDataTypeStr=boolean  ZeroCross=off
  Data Store Read Error : DataStoreRead  DataStoreName=Error  SampleTime=Ts
  Data Store Read Force Sensor : DataStoreRead  DataStoreName=Force_sensor  SampleTime=Ts
  Data Store Read Force Sensor_ : DataStoreRead  DataStoreName=Force_sensor
  Data Store Read No WorkSpace_ : DataStoreRead  DataStoreName=X_CONTAINER  SampleTime=Ts
  Data Store Read No WorkSpace__ : DataStoreRead  DataStoreName=X_CONTAINER  SampleTime=Ts
  Data Store Read No Worspace : DataStoreRead  DataStoreName=No_WorkSpace  SampleTime=Ts
  Data Store Read Pos x_y : DataStoreRead  DataStoreName=Pos_x_y
  Data Store Read Z high : DataStoreRead  DataStoreName=Z_HIGH  SampleTime=Ts
  Distance_y_table : Constant  Value=19
  Distance_z_table : Constant  Value=11.5
  Logical Operator{,2,5..6,8} (5 alike) : Logic  AllPortsSameDT=off  OutDataTypeStr=boolean
  Logical Operator1 : Logic  Operator=NOT  AllPortsSameDT=off  OutDataTypeStr=boolean
  Logical Operator4 : Logic  Operator=NOT  AllPortsSameDT=off  OutDataTypeStr=boolean
  Logical Operator7 : Logic  Operator=NOT  AllPortsSameDT=off  OutDataTypeStr=boolean
  PHI_FIX : Constant  Value=-90
  Switch{,1..2,4..10} (10 alike) : Switch  Threshold=1  ZeroCross=off
  X_FIX : Constant  Value=-26
  X_I : Constant  Value=-25
  Y_FIX : Constant  Value=17
  Z_CAM : Constant  Value=3
  Z_FIX : Constant  Value=3
  Z_I : Constant  Value=31
  Z_high : Constant  Value=42.5
  X_CAMARA : Outport
  X_FIXED : Outport  Port=2
  Y_CAMARA : Outport  Port=3
  Y_FIXED : Outport  Port=4
  Z_CAMARA : Outport  Port=5
  Z_FIXED : Outport  Port=6
  PHI_CAMARA : Outport  Port=7
  PHI_FIXED : Outport  Port=8
  wires:
  Logical Operator4/1 -> Abertura_sensor/1
  PHI_FIX/1 -> PHI_FIXED/1, PHI_CAMARA/1
  Compare To Constant2/1 -> Logical Operator/2
  Switch/1 -> X_CAMARA/1
  X_I/1 -> Switch/1
  Logical Operator/1 -> Logical Operator4/1, Switch2/2, Switch/2, Switch1/2
  Compare To Constant/1 -> Logical Operator/1
  Z_I/1 -> Switch4/3, Switch2/1, Switch5/1
  Y_CAM/1 -> Add2/1, Compare To Constant/1
  X_CAM/1 -> Compare To Constant2/1, Switch/3, Switch6/3
  Z_FIX/1 -> Add/2
  Distance_z_table/1 -> Add1/2, Add/1
  Add1/1 -> Z_CAMARA/1
  Switch1/1 -> Y_CAMARA/1
  Add2/1 -> Switch7/3, Switch1/3
  Switch4/1 -> Switch2/3
  Z_CAM/1 -> Switch4/1
  Switch2/1 -> Switch5/3
  Switch5/1 -> Add1/1
  X_FIX/1 -> Switch6/1, Switch9/1
  Z_high/1 -> Switch8/1
  Add/1 -> Switch8/3
  Switch8/1 -> Z_FIXED/1
  Switch6/1 -> Switch9/3
  Switch9/1 -> X_FIXED/1
  Switch10/1 -> Y_FIXED/1
  Switch7/1 -> Switch10/3
  Data Store Read No WorkSpace__/1 -> Switch9/2, Switch10/2
  Data Store Read No Worspace/1 -> Logical Operator1/1
  Logical Operator1/1 -> Logical Operator2/2
  Data Store Read Error/1 -> Logical Operator2/1
  Logical Operator2/1 -> Switch4/2
  Logical Operator5/1 -> Switch7/2, Switch6/2
  Data Store Read Z high/1 -> Logical Operator5/1
  Data Store Read Force Sensor/1 -> Logical Operator5/2
  Data Store Read No WorkSpace_/1 -> Logical Operator7/1
  Logical Operator7/1 -> Logical Operator6/2
  Data Store Read Force Sensor_/1 -> Logical Operator8/2, Logical Operator6/1
  Logical Operator6/1 -> Switch8/2
  Data Store Read Pos x_y/1 -> Logical Operator8/1
  Logical Operator8/1 -> Switch5/2
  Y_FIX/1 -> Switch7/1, Switch10/1, Switch1/1
  Distance_y_table/1 -> Add2/2

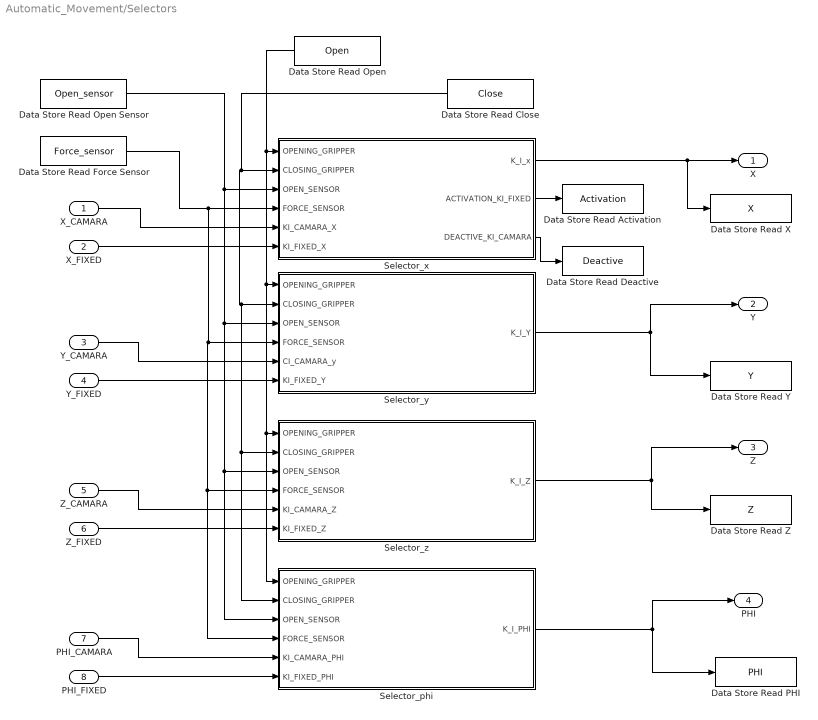
== system Automatic_Movement/Selectors ==
  X_CAMARA : Inport
  X_FIXED : Inport  Port=2
  Y_CAMARA : Inport  Port=3
  Y_FIXED : Inport  Port=4
  Z_CAMARA : Inport  Port=5
  Z_FIXED : Inport  Port=6
  PHI_CAMARA : Inport  Port=7
  PHI_FIXED : Inport  Port=8
  " Data Store Read X" : DataStoreWrite  DataStoreName=X  SampleTime=Ts
  Data Store Read Close : DataStoreRead  DataStoreName=Close  SampleTime=Ts
  Data Store Read Force Sensor : DataStoreRead  DataStoreName=Force_sensor  SampleTime=Ts
  Data Store Read Open : DataStoreRead  DataStoreName=Open  SampleTime=Ts
  Data Store Read Open Sensor : DataStoreRead  DataStoreName=Open_sensor  SampleTime=Ts
  "Data Store Read Activation " : DataStoreWrite  DataStoreName=Activation  SampleTime=Ts
  Data Store Read Deactive : DataStoreWrite  DataStoreName=Deactive  SampleTime=Ts
  "Data Store Read PHI " : DataStoreWrite  DataStoreName=PHI  SampleTime=Ts
  "Data Store Read Y " : DataStoreWrite  DataStoreName=Y  SampleTime=Ts
  "Data Store Read Z " : DataStoreWrite  DataStoreName=Z  SampleTime=Ts
  Selector_phi : Subsystem
  Selector_x : Subsystem
  Selector_y : Subsystem
  Selector_z : Subsystem
  "X " : Outport
  Y : Outport  Port=2
  Z : Outport  Port=3
  PHI : Outport  Port=4
  wires:
  Selector_x/2(ACTIVATION_KI_FIXED) -> "Data Store Read Activation "/1
  Selector_z/1(K_I_Z) -> Z/1, "Data Store Read Z "/1
  Selector_x/1(K_I_x) -> " Data Store Read X"/1, "X "/1
  Selector_phi/1(K_I_PHI) -> "Data Store Read PHI "/1, PHI/1
  Selector_y/1(K_I_Y) -> "Data Store Read Y "/1, Y/1
  Data Store Read Open Sensor/1 -> Selector_phi/3(OPEN_SENSOR), Selector_z/3(OPEN_SENSOR), Selector_y/3(OPEN_SENSOR), Selector_x/3(OPEN_SENSOR)
  X_CAMARA/1 -> Selector_x/5(KI_CAMARA_X)
  Y_FIXED/1 -> Selector_y/6(KI_FIXED_Y)
  Z_FIXED/1 -> Selector_z/6(KI_FIXED_Z)
  X_FIXED/1 -> Selector_x/6(KI_FIXED_X)
  Z_CAMARA/1 -> Selector_z/5(KI_CAMARA_Z)
  Y_CAMARA/1 -> Selector_y/5(CI_CAMARA_y)
  PHI_FIXED/1 -> Selector_phi/6(KI_FIXED_PHI)
  PHI_CAMARA/1 -> Selector_phi/5(KI_CAMARA_PHI)
  Data Store Read Close/1 -> Selector_phi/2(CLOSING_GRIPPER), Selector_z/2(CLOSING_GRIPPER), Selector_y/2(CLOSING_GRIPPER), Selector_x/2(CLOSING_GRIPPER)
  Data Store Read Open/1 -> Selector_phi/1(OPENING_GRIPPER), Selector_z/1(OPENING_GRIPPER), Selector_y/1("OPENING_GRIPPER "), Selector_x/1(OPENING_GRIPPER)
  Data Store Read Force Sensor/1 -> Selector_phi/4(FORCE_SENSOR), Selector_z/4(FORCE_SENSOR), Selector_y/4(FORCE_SENSOR), Selector_x/4(FORCE_SENSOR)
  Selector_x/3(DEACTIVE_KI_CAMARA) -> Data Store Read Deactive/1

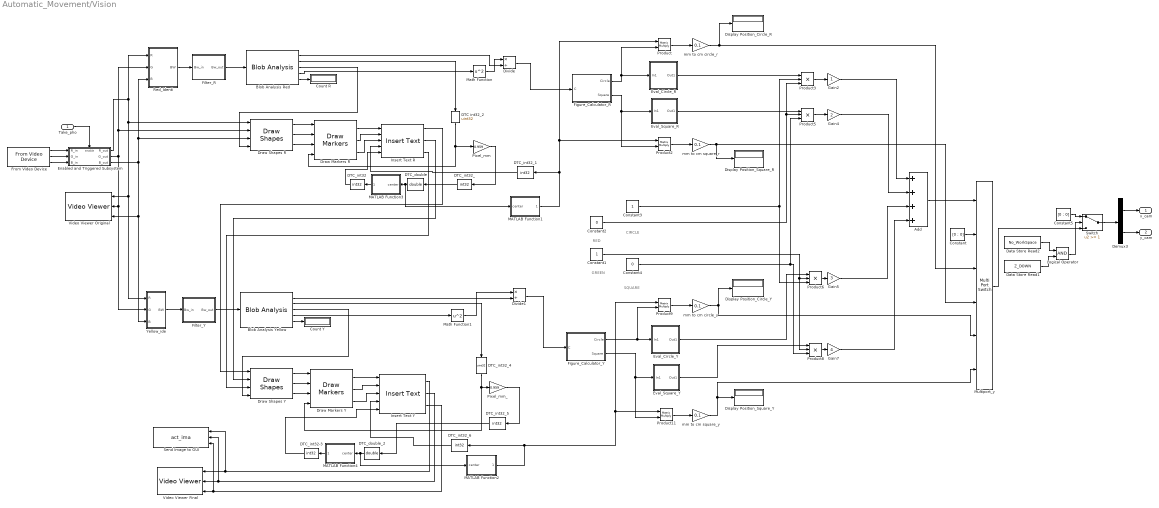
== system Automatic_Movement/Vision ==
  note: GREEN
  note: RED
  note: SQUARE
  note: CIRCLE
  Take_pho : Inport
  Add : Sum  Inputs=++++
  Blob Analysis Red : visionstatistics/Blob Analysis  Tag=vipblks_row_conv  area=on  centroid=on  bBox=on  majorAxis=off  minorAxis=off  angle=off  eccentricity=off  equivDiameterSq=off  extent=off  perimeter=on  maxBlobs=2  warnIfNumBlobsExceeded=on  isCount=on  useMinArea=on  minArea=700  useMaxArea=off  maxArea=intmax('uint32')  excludeBorderBlob=on  outDT=double  isOutVarDim=off  isFill=on  fillValues=-1  conn=8  isLabel=off  outputMode=Binary point scaling  outputWordLength=32  outputFracLength=16  firstCoeffMode=Binary point scaling  firstCoeffWordLength=16  firstCoeffFracLength=14  secondCoeffMode=Binary point scaling  secondCoeffWordLength=32  secondCoeffFracLength=16  accumMode=Binary point scaling  accumWordLength=32  accumFracLength=0  prodOutputMode=Binary point scaling  prodOutputWordLength=32  prodOutputFracLength=16  roundingMode=Floor  overflowMode=off
  Blob Analysis Yellow : visionstatistics/Blob Analysis  Tag=vipblks_row_conv  area=on  centroid=on  bBox=on  majorAxis=off  minorAxis=off  angle=off  eccentricity=off  equivDiameterSq=off  extent=off  perimeter=on  maxBlobs=2  warnIfNumBlobsExceeded=on  isCount=on  useMinArea=on  minArea=700  useMaxArea=off  maxArea=intmax('uint32')  excludeBorderBlob=on  outDT=double  isOutVarDim=off  isFill=on  fillValues=-1  conn=8  isLabel=off  outputMode=Binary point scaling  outputWordLength=32  outputFracLength=16  firstCoeffMode=Binary point scaling  firstCoeffWordLength=16  firstCoeffFracLength=14  secondCoeffMode=Binary point scaling  secondCoeffWordLength=32  secondCoeffFracLength=16  accumMode=Binary point scaling  accumWordLength=32  accumFracLength=0  prodOutputMode=Binary point scaling  prodOutputWordLength=32  prodOutputFracLength=16  roundingMode=Floor  overflowMode=off
  Constant : Constant  Value=[0 ; 0]
  Constant1 : Constant
  Constant2 : Constant  Value=0
  Constant3 : Constant
  Constant4 : Constant  Value=0
  Constant5 : Constant  Value=[0 ; 0]
  Count R : Display
  Count Y : Display
  DTC int32_2 : DataTypeConversion  OutDataTypeStr=uint32
  DTC_double : DataTypeConversion  OutDataTypeStr=double
  DTC_double_2 : DataTypeConversion  OutDataTypeStr=double
  DTC_int32 : DataTypeConversion  OutDataTypeStr=int32
  DTC_int32-3 : DataTypeConversion  OutDataTypeStr=int32
  DTC_int32_{,1,5..6} (4 alike) : DataTypeConversion  OutDataTypeStr=int32
  DTC_int32_4 : DataTypeConversion  OutDataTypeStr=uint32
  Data Store Read1 : DataStoreRead  DataStoreName=Z_DOWN
  Data Store Read2 : DataStoreRead  DataStoreName=No_WorkSpace
  Demux3 : Demux  Outputs=2
  Display Position_Circle_R : Display
  Display Position_Circle_Y : Display
  Display Position_Square_R : Display
  Display Position_Square_Y : Display
  Divide : Product  Inputs=*/
  Divide1 : Product  Inputs=*/
  Draw Markers R : visiontextngfix/Draw Markers  shape=Plus  size=8  fill=off  fillClrSource=Specify via dialog  display=User-specified value  intensity=200  color=[0 0 1]  opacity=0.6  viewport=Entire image  antialiasing=off  inType=Obsolete  imagePorts=Separate color signals  prodOutputMode=Binary point scaling  prodOutputWordLength=32  prodOutputFracLength=14  memoryMode=Specify word length  memoryWordLength=16  memoryFracLength=15  roundingMode=Floor  overflowMode=off
  Draw Markers Y : visiontextngfix/Draw Markers  shape=Plus  size=8  fill=off  fillClrSource=Specify via dialog  display=User-specified value  intensity=200  color=[0 0 1]  opacity=0.6  viewport=Entire image  antialiasing=off  inType=Obsolete  imagePorts=Separate color signals  prodOutputMode=Binary point scaling  prodOutputWordLength=32  prodOutputFracLength=14  memoryMode=Specify word length  memoryWordLength=16  memoryFracLength=15  roundingMode=Floor  overflowMode=off
  Draw Shapes R : visiontextngfix/Draw Shapes  shape=Rectangles  fill=off  lineWidth=1  fillClrSource=Specify via dialog  display=User-specified value  intensity=200  color=[0 0 255]  opacity=0.5  viewport=Entire image  antialiasing=off  inType=Obsolete  imagePorts=Separate color signals  prodOutputMode=Binary point scaling  prodOutputWordLength=32  prodOutputFracLength=14  memoryMode=Specify word length  memoryWordLength=16  memoryFracLength=14  roundingMode=Floor  overflowMode=off
  Draw Shapes Y : visiontextngfix/Draw Shapes  shape=Rectangles  fill=off  lineWidth=1  fillClrSource=Specify via dialog  display=User-specified value  intensity=200  color=[0 0 255]  opacity=0.5  viewport=Entire image  antialiasing=off  inType=Obsolete  imagePorts=Separate color signals  prodOutputMode=Binary point scaling  prodOutputWordLength=32  prodOutputFracLength=14  memoryMode=Specify word length  memoryWordLength=16  memoryFracLength=14  roundingMode=Floor  overflowMode=off
  Enabled and Triggered Subsystem : Subsystem  TreatAsAtomicUnit=on
  Eval_Circle_R : Subsystem
  Eval_Circle_Y : Subsystem
  Eval_Square_R : Subsystem
  Eval_Square_Y : Subsystem
  Figure_Calculator_R : Subsystem
  Figure_Calculator_Y : Subsystem
  Filter_R : Subsystem
  Filter_Y : Subsystem
  From Video Device : imaqlib/From Video Device  DeviceMenu=(none)  Device=winvideo 1 (Logitech HD Webcam C525)  ObjConstructor=videoinput('winvideo', 1)  VideoFormatMenu=(none)  VideoFormat=RGB24_640x480  VideoSource=input1  ROIPosition=[184 115 146 417]  EnableHWTrigger=off  TriggerConfiguration=none/none  SampleTime=1/5  OutputPortsMode=Separate color signals  DataType=single  CanDoHWTrigger=no  ReturnedColorSpace=rgb  BlockHandle=645.0004  ROIWidth=417  ROIHeight=146  ROIColumn=115  ROIRow=184  EngXMLPath=C:\Program Files\MATLAB\R2017a\toolbox\imaq\imaq\private  DevXMLPath=C:\ProgramData\MATLAB\SupportPackages\R2017a\toolbox\imaq\supportpackages\genericvideo\adaptor\win64  EngLibPath=C:\Program Files\MATLAB\R2017a\toolbox\imaq\imaqblks\imaqmex\win64  ColorSpace=rgb  BayerSensorAlignment=grbg
  Gain2 : Gain
  Gain4 : Gain  Gain=2
  Gain5 : Gain  Gain=3
  Gain7 : Gain  Gain=4
  Insert Text R : visiontextngfix/Insert Text  inputType=Obsolete  theText='[%i;%i]'  getTextLocFrom=Input port  textLoc=[1 1]  getTextColorFrom=Specify via dialog  textColor=[0 0 0]  getTextIntensityFrom=Specify via dialog  textIntensity=0  getTextOpacityFrom=Specify via dialog  textOpacity=1  dummyVar2=0  dummyVar3=0  dummyVar4=0  imagePorts=Separate color signals  isInputTransposed=off  fontFace=Calibri  dummyVar1=0  blockFontSize=20  antiAliased=on
  Insert Text Y : visiontextngfix/Insert Text  inputType=Obsolete  theText='[%i;%i]'  getTextLocFrom=Input port  textLoc=[1 1]  getTextColorFrom=Specify via dialog  textColor=[0 0 0]  getTextIntensityFrom=Specify via dialog  textIntensity=0  getTextOpacityFrom=Specify via dialog  textOpacity=1  dummyVar2=0  dummyVar3=0  dummyVar4=0  imagePorts=Separate color signals  isInputTransposed=off  fontFace=Calibri  dummyVar1=0  blockFontSize=20  antiAliased=on
  Logical Operator : Logic  AllPortsSameDT=off  OutDataTypeStr=boolean
  MATLAB Function1 : MATLAB Function  TreatAsAtomicUnit=on
      settings: PermitHierarchicalResolution=ParametersOnly
  MATLAB Function2 : MATLAB Function  TreatAsAtomicUnit=on
      settings: PermitHierarchicalResolution=ParametersOnly
  MATLAB Function3 : MATLAB Function  TreatAsAtomicUnit=on
      settings: PermitHierarchicalResolution=ParametersOnly
  MATLAB Function4 : MATLAB Function  TreatAsAtomicUnit=on
      settings: PermitHierarchicalResolution=ParametersOnly
  Math Function : Math  Operator=square  SaturateOnIntegerOverflow=on
  Math Function1 : Math  Operator=square  SaturateOnIntegerOverflow=on
  Multiport_y : MultiPortSwitch  DataPortOrder=Specify indices  Inputs=6  DataPortIndices={0,1,2,3,4}  DiagnosticForDefault=None
  Pixel_mm : Gain  Gain=0.959
  Pixel_mm_ : Gain  Gain=0.959
  Product{,2,9,11} (4 alike) : Product  Multiplication=Matrix(*)
  Product{3,5..6,8} (4 alike) : Product  Inputs=3
  Red_Identi : Subsystem
  Send Image to GUI : M-S-Function  FunctionName=act_ima
  Switch : Switch  Threshold=1  ZeroCross=off
  Video Viewer Final : visionsinks/Video Viewer  inputType=Obsolete7b  useColorMap=off  colormapValue=gray(256)  specRange=off  minInputVal=0  maxInputVal=255  FigPos=[476 894 766 716]  AxisZoom=on  trueSizedOnce=off  OpenAtMdlStart=off  imagePorts=separate color signals
  Video Viewer Original : visionsinks/Video Viewer  inputType=Obsolete7b  useColorMap=off  colormapValue=gray(256)  specRange=off  minInputVal=0  maxInputVal=255  FigPos=[1 822 1444 724]  AxisZoom=on  trueSizedOnce=off  OpenAtMdlStart=off  imagePorts=separate color signals
  Yellow_ide : Subsystem
  mm to cm circle_r : Gain  Gain=0.1
  mm to cm circle_y : Gain  Gain=0.1
  mm to cm square_r : Gain  Gain=0.1
  mm to cm square_y : Gain  Gain=0.1
  x_cam : Outport
  y_cam : Outport  Port=2
  wires:
  Blob Analysis Red/5 -> Count R/1
  mm to cm circle_r/1 -> Multiport_y/3, Display Position_Circle_R/1
  Enabled and Triggered Subsystem/3(B_out) -> Red_Identi/3(B), Draw Shapes R/3, Yellow_ide/3(B), Video Viewer Original/3
  Eval_Circle_R/1(Out1) -> Product3/1
  Product6/1 -> Gain5/1
  Draw Markers R/3 -> Insert Text R/3
  Math Function/1 -> Divide/1
  Gain4/1 -> Add/2
  Constant2/1 -> Product3/3, Product5/2
  Figure_Calculator_R/2(Square) -> Product2/2, Eval_Square_R/1(In1)
  Draw Markers R/1 -> Insert Text R/1
  Enabled and Triggered Subsystem/1(R_out) -> Red_Identi/1(R), Draw Shapes R/1, Yellow_ide/1(R), Video Viewer Original/1
  MATLAB Function1/1(variable) -> DTC_int32_1/1, Product2/1, Product/1
  Product/1 -> mm to cm circle_r/1
  Blob Analysis Red/4 -> Math Function/1
  Take_pho/1 -> Enabled and Triggered Subsystem/Enable
  Product3/1 -> Gain2/1
  Product2/1 -> mm to cm square_r/1
  Gain7/1 -> Add/4
  Insert Text R/2 -> Draw Shapes Y/2
  Figure_Calculator_R/1(Circle) -> Product/2, Eval_Circle_R/1(In1)
  Constant4/1 -> Product8/3, Product5/3
  Draw Shapes R/1 -> Draw Markers R/1
  Constant3/1 -> Product6/3, Product3/2
  Gain2/1 -> Add/1
  Draw Markers R/2 -> Insert Text R/2
  Eval_Square_R/1(Out1) -> Product5/1
  Enabled and Triggered Subsystem/2(G_out) -> Red_Identi/2(G), Draw Shapes R/2, Yellow_ide/2(G), Video Viewer Original/2
  Product8/1 -> Gain7/1
  Product5/1 -> Gain4/1
  Draw Shapes R/2 -> Draw Markers R/2
  DTC int32_2/1 -> Pixel_mm/1, Draw Markers R/4
  Divide/1 -> Figure_Calculator_R/1("C ")
  Insert Text R/1 -> Draw Shapes Y/1
  Insert Text R/3 -> Draw Shapes Y/3
  Constant1/1 -> Product8/2, Product6/2
  Draw Shapes R/3 -> Draw Markers R/3
  Blob Analysis Red/1 -> Divide/2
  DTC_int32_1/1 -> Insert Text R/4
  From Video Device/1 -> Enabled and Triggered Subsystem/1(R_in)
  Pixel_mm/1 -> DTC_int32_/1
  DTC_double/1 -> MATLAB Function1/1(center), MATLAB Function3/1(center)
  Blob Analysis Red/2 -> DTC int32_2/1
  Gain5/1 -> Add/3
  DTC_int32_/1 -> DTC_double/1
  Blob Analysis Red/3 -> Draw Shapes R/4
  From Video Device/3 -> Enabled and Triggered Subsystem/3(B_in)
  From Video Device/2 -> Enabled and Triggered Subsystem/2(G_in)
  Add/1 -> Multiport_y/1
  Demux3/2 -> y_cam/1
  Demux3/1 -> x_cam/1
  Red_Identi/1(BW) -> Filter_R/1(Bw_in)
  Filter_R/1(Bw_out) -> Blob Analysis Red/1
  mm to cm square_r/1 -> Multiport_y/4, Display Position_Square_R/1
  Filter_Y/1(Bw_out) -> Blob Analysis Yellow/1
  Insert Text Y/1 -> Send Image to GUI/1, Video Viewer Final/1
  Draw Shapes Y/3 -> Draw Markers Y/3
  Figure_Calculator_Y/1(Circle) -> Product9/2, Eval_Circle_Y/1(In1)
  Insert Text Y/2 -> Send Image to GUI/2, Video Viewer Final/2
  Product11/1 -> mm to cm square_y/1
  Draw Markers Y/2 -> Insert Text Y/2
  Draw Shapes Y/1 -> Draw Markers Y/1
  Eval_Square_Y/1(Out1) -> Product8/1
  DTC_double_2/1 -> MATLAB Function2/1(center), MATLAB Function4/1(center)
  Blob Analysis Yellow/4 -> Math Function1/1
  DTC_int32_4/1 -> Draw Markers Y/4, Pixel_mm_/1
  Draw Shapes Y/2 -> Draw Markers Y/2
  MATLAB Function2/1(variable) -> Product11/1, Product9/1, DTC_int32_6/1
  DTC_int32_6/1 -> Insert Text Y/4
  mm to cm square_y/1 -> Multiport_y/6, Display Position_Square_Y/1
  Divide1/1 -> Figure_Calculator_Y/1("C ")
  Eval_Circle_Y/1(Out1) -> Product6/1
  Math Function1/1 -> Divide1/1
  Blob Analysis Yellow/2 -> DTC_int32_4/1
  Figure_Calculator_Y/2(Square) -> Product11/2, Eval_Square_Y/1(In1)
  DTC_int32_5/1 -> DTC_double_2/1
  Draw Markers Y/3 -> Insert Text Y/3
  Draw Markers Y/1 -> Insert Text Y/1
  Blob Analysis Yellow/3 -> Draw Shapes Y/4
  Product9/1 -> mm to cm circle_y/1
  Blob Analysis Yellow/1 -> Divide1/2
  Insert Text Y/3 -> Send Image to GUI/3, Video Viewer Final/3
  Blob Analysis Yellow/5 -> Count Y/1
  Pixel_mm_/1 -> DTC_int32_5/1
  Yellow_ide/1(BW) -> Filter_Y/1(Bw_in)
  mm to cm circle_y/1 -> Multiport_y/5, Display Position_Circle_Y/1
  Switch/1 -> Demux3/1
  Data Store Read2/1 -> Logical Operator/1
  Data Store Read1/1 -> Logical Operator/2
  Multiport_y/1 -> Switch/3
  Constant/1 -> Multiport_y/2
  Constant5/1 -> Switch/1
  Logical Operator/1 -> Switch/2
  MATLAB Function3/1(location) -> DTC_int32/1
  DTC_int32/1 -> Insert Text R/5
  MATLAB Function4/1(location) -> DTC_int32-3/1
  DTC_int32-3/1 -> Insert Text Y/5
